simulink model "TwoLink_mdl"  (R2018b)
settings: Solver=ode15s  StartTime=0.0  StopTime=20  MaxStep=0.01  RelTol=1e-5  EnableMultiTasking=on
values from neighbouring files (symbols this model uses):
  Dp = diag([0 0 0.09 0.05])    [TwoLink_nl.m]    (also in TwoLink_pwa.m)
  F = [eye(2);zeros(2)]    [TwoLink_nl.m]    (also in TwoLink_pwa.m)
  K = diag([0 0 89.1473 45.6434])    [TwoLink_nl.m]    (also in TwoLink_pwa.m)
  M_pi = [17.0296  0.8856  9.7776  0.8430 ... (first row only)    [TwoLink_nl.m]    (also in TwoLink_pwa.m)
  M_pi2 = [34.7077  9.7246 23.6398  5.9114 ... (first row only)    [TwoLink_nl.m]    (also in TwoLink_pwa.m)
  p0 = pi/2    (= 1.57079632679)    [TwoLink_pwa.m]
libraries: lpvlibrary x2
settings Model: Creator=Fernando  LastModifiedBy=ferna
settings OptimizationCC: LifeSpan=inf
settings DebuggingCC: SFUnexpectedBacktrackingDiag=warning  SFNoUnconditionalDefaultTransitionDiag=warning
settings SFSimCC: SimUseLocalCustomCode=off
settings RTWCC: RTWUseLocalCustomCode=off
settings CodeAppCC: StateflowObjectComments=on
settings GRTTargetCC: TargetLangStandard=C89/C90 (ANSI)  GeneratePreprocessorConditionals=Disable all
settings ConfigComp: CovMetricSettings=dw  CovHtmlReporting=on  CovSaveCumulativeToWorkspaceVar=on  CovSaveSingleToWorkspaceVar=on  CovExternalEMLEnable=off

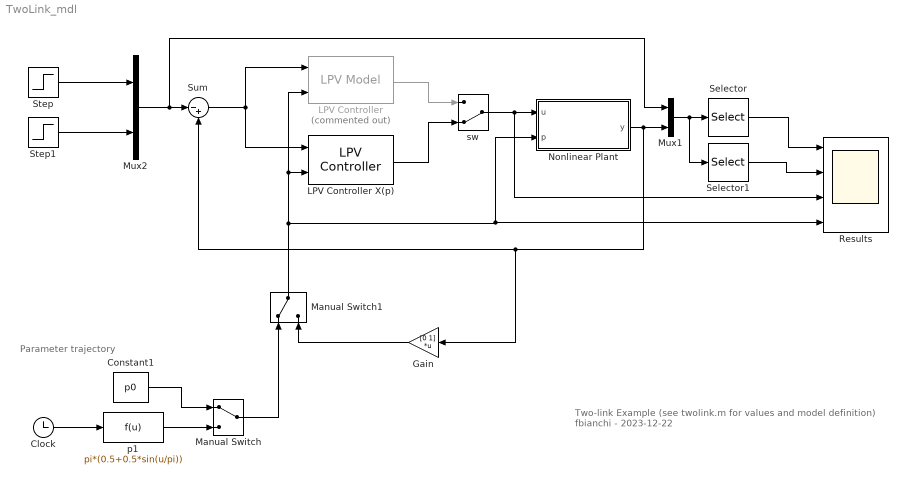
== system TwoLink_mdl ==
  note: Parameter trajectory
  note: Two-link Example
      | (see twolink.m for values and model definition)
      | fbianchi - 2023-12-22
  Clock : Clock
  Constant1 : Constant  Value=p0
  Gain : Gain  Gain=[0 1]  Multiplication=Matrix(K*u)
  LPV Controller : lpvlibrary/LPV Model  Commented=on  pdG=pdK  x0=0
      settings: SourceProductName=LPV Toolbox
  LPV Controller X(p) : lpvlibrary/LPV Controller  pdK=pdK  x0=0
      settings: SourceProductName=LPV Toolbox
  Manual Switch : ManualSwitch
  Manual Switch1 : ManualSwitch
  Mux1 : Mux  Inputs=[2 2]
  Mux2 : Mux  Inputs=2
  Nonlinear Plant : Subsystem
  Results : Scope  NumInputPorts=4
  Selector : Selector  InputPortWidth=4  IndexOptions=Index vector (dialog)  Indices=[1 3]  OutputSizes=1
  Selector1 : Selector  InputPortWidth=4  IndexOptions=Index vector (dialog)  Indices=[2 4]  OutputSizes=1
  Step : Step  SampleTime=0
  Step1 : Step  SampleTime=0
  Sum : Sum  Inputs=|-+
  p1 : Fcn  Expr=pi*(0.5+0.5*sin(u/pi))
  sw : ManualSwitch  CurrentSetting=0
  wires:
  Sum/1 -> LPV Controller X(p)/1, LPV Controller/1
  Mux2/1 -> Sum/1, Mux1/1
  Mux1/1 -> Selector/1, Selector1/1
  Selector/1 -> Results/1
  Selector1/1 -> Results/2
  Clock/1 -> p1/1
  Constant1/1 -> Manual Switch/1
  p1/1 -> Manual Switch/2
  Step/1 -> Mux2/1
  Step1/1 -> Mux2/2
  Nonlinear Plant/1(y) -> Gain/1, Sum/2, Mux1/2
  sw/1 -> Results/3, Nonlinear Plant/1(u)
  LPV Controller/1 -> sw/1
  LPV Controller X(p)/1 -> sw/2
  Manual Switch1/1 -> Nonlinear Plant/2(p), Results/4, LPV Controller/2, LPV Controller X(p)/2
  Manual Switch/1 -> Manual Switch1/1
  Gain/1 -> Manual Switch1/2

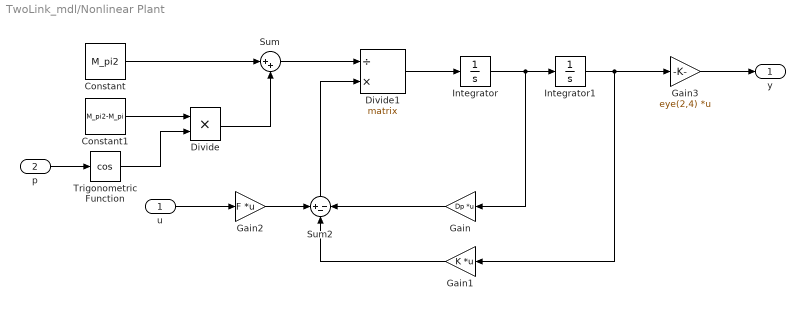
== system TwoLink_mdl/Nonlinear Plant ==
  u : Inport
  p : Inport  Port=2
  Constant : Constant  Value=M_pi2
  Constant1 : Constant  Value=M_pi2-M_pi
  Divide : Product  Inputs=**
  Divide1 : Product  Inputs=/*  Multiplication=Matrix(*)
  Gain : Gain  Gain=Dp  Multiplication=Matrix(K*u)
  Gain1 : Gain  Gain=K  Multiplication=Matrix(K*u)
  Gain2 : Gain  Gain=F  Multiplication=Matrix(K*u)
  Gain3 : Gain  Gain=eye(2,4)  Multiplication=Matrix(K*u)
  Integrator : Integrator  InitialCondition=zeros(4,1)
  Integrator1 : Integrator  InitialCondition=zeros(4,1)
  Sum : Sum  Inputs=|++
  Sum2 : Sum  Inputs=+--
  Trigonometric Function : Trigonometry  Operator=cos
  y : Outport
  wires:
  Gain/1 -> Sum2/3
  Constant/1 -> Sum/1
  Gain1/1 -> Sum2/2
  Trigonometric Function/1 -> Divide/2
  Integrator1/1 -> Gain3/1, Gain1/1
  Divide/1 -> Sum/2
  Constant1/1 -> Divide/1
  Integrator/1 -> Gain/1, Integrator1/1
  u/1 -> Gain2/1
  Sum2/1 -> Divide1/2
  Divide1/1 -> Integrator/1
  Sum/1 -> Divide1/1
  Gain2/1 -> Sum2/1
  p/1 -> Trigonometric Function/1
  Gain3/1 -> y/1
